simulink subsystem "Plant"  (R2024b)
settings: Solver=VariableStepAuto  StartTime=0.0  StopTime=10.0  RelTol=1e-3
undefined symbols (not defined in the file): fast, GenEff, matches, OutList, rpm2radps, strmatch, TMax
libraries: simulink_extras x1
settings Model: Creator=jhummel  LastModifiedBy=jhummel
settings ModelReferenceCC: EnableRefExpFcnMdlSchedulingChecks=on
settings RTWCC: GPUComputeCapability=3.5

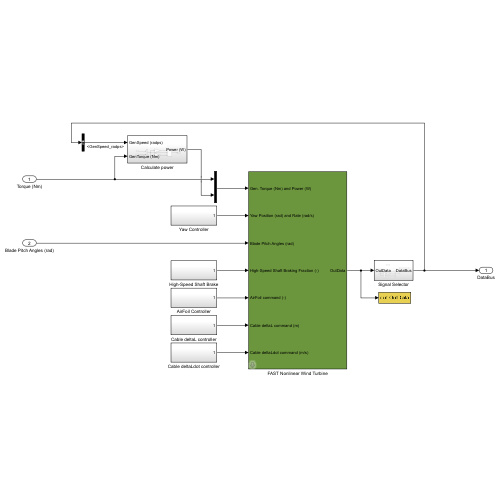
[thumbnail: Simulink's stored preview of the top-level diagram]
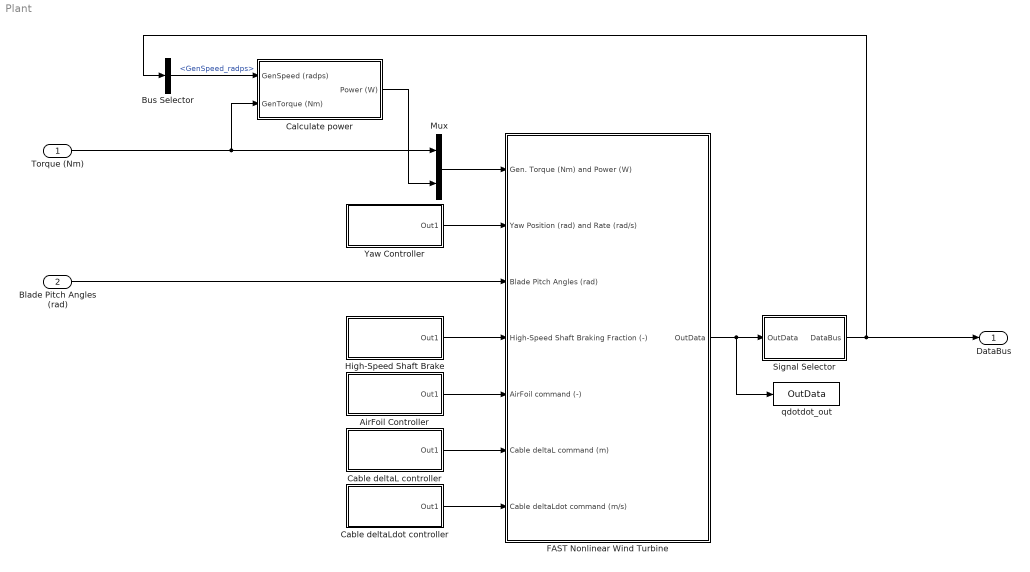
== system Plant ==
  Torque (Nm) : Inport
  Blade Pitch Angles (rad) : Inport  Port=2
  AirFoil Controller : Subsystem
  Bus Selector : BusSelector  OutputSignals=GenSpeed_radps
  Cable deltaL controller : Subsystem
  Cable deltaLdot controller : Subsystem
  Calculate power : Subsystem
  FAST Nonlinear Wind Turbine : Subsystem  mask(FAST Nonlinear Wind Turbine){}
      mask help: This block contains the FAST S-Function.
      mask init:
      | clear FAST_SFunc
  High-Speed Shaft Brake : Subsystem
  Mux : Mux  Inputs=2
  Signal Selector : Subsystem
  Yaw Controller : Subsystem
  qdotdot_out : ToWorkspace  VariableName=OutData  SampleTime=-1
  DataBus : Outport
  wires:
  Yaw Controller/1(Out1) -> FAST Nonlinear Wind Turbine/2(Yaw Position (rad) and Rate (rad/s))
  Mux/1 -> FAST Nonlinear Wind Turbine/1(Gen. Torque (Nm) and Power (W))
  Cable deltaL controller/1(Out1) -> FAST Nonlinear Wind Turbine/6(Cable deltaL command (m))
  High-Speed Shaft Brake/1(Out1) -> FAST Nonlinear Wind Turbine/4(High-Speed Shaft Braking Fraction (-))
  AirFoil Controller/1(Out1) -> FAST Nonlinear Wind Turbine/5(AirFoil command (-))
  Signal Selector/1(DataBus) -> Bus Selector/1, DataBus/1
  Calculate power/1(Power (W)) -> Mux/2
  Torque (Nm)/1 -> Calculate power/2(GenTorque (Nm)), Mux/1
  Cable deltaLdot controller/1(Out1) -> FAST Nonlinear Wind Turbine/7(Cable deltaLdot command (m/s))
  Bus Selector/1 -> Calculate power/1(GenSpeed (radps))  "<GenSpeed_radps>"
  FAST Nonlinear Wind Turbine/1(OutData) -> Signal Selector/1(OutData), qdotdot_out/1
  Blade Pitch Angles (rad)/1 -> FAST Nonlinear Wind Turbine/3(Blade Pitch Angles (rad))

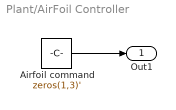
== system Plant/AirFoil Controller ==
  Airfoil command : Constant  Value=zeros(1,3)'
  Out1 : Outport
  wires:
  Airfoil command/1 -> Out1/1

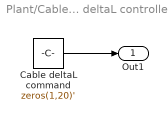
== system Plant/Cable deltaL controller ==
  Cable deltaL command : Constant  Value=zeros(1,20)'
  Out1 : Outport
  wires:
  Cable deltaL command/1 -> Out1/1

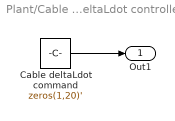
== system Plant/Cable deltaLdot controller ==
  Cable deltaLdot command : Constant  Value=zeros(1,20)'
  Out1 : Outport
  wires:
  Cable deltaLdot command/1 -> Out1/1

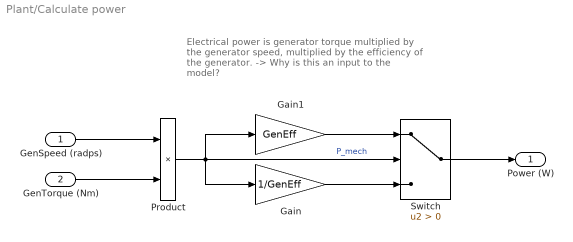
== system Plant/Calculate power ==
  note: Electrical power is generator torque multiplied by the generator speed, multiplied by the efficiency of the generator.
      | -> Why is this an input to the model?
  GenSpeed (radps) : Inport
  GenTorque (Nm) : Inport  Port=2
  Gain : Gain  Gain=1/GenEff
  Gain1 : Gain  Gain=GenEff
  Product : Product
  Switch : Switch  Criteria=u2 > Threshold  SaturateOnIntegerOverflow=off  InputSameDT=off
  Power (W) : Outport
  wires:
  Gain/1 -> Switch/3
  Product/1 -> Switch/2, Gain/1, Gain1/1  "P_mech"
  Gain1/1 -> Switch/1
  GenTorque (Nm)/1 -> Product/2
  GenSpeed (radps)/1 -> Product/1
  Switch/1 -> Power (W)/1

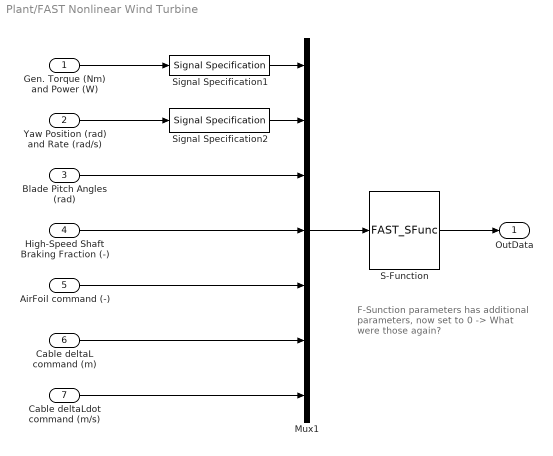
== system Plant/FAST Nonlinear Wind Turbine ==
  note: F-Sunction parameters has additional parameters, now set to 0 -> What were those again?
  Gen. Torque (Nm) and Power (W) : Inport
  Yaw Position (rad) and Rate (rad/s) : Inport  Port=2
  Blade Pitch Angles (rad) : Inport  Port=3
  High-Speed Shaft Braking Fraction (-) : Inport  Port=4
  AirFoil command (-) : Inport  Port=5
  Cable deltaL command (m) : Inport  Port=6
  Cable deltaLdot command (m/s) : Inport  Port=7
  Mux1 : Mux  Inputs=7
  S-Function : S-Function  FunctionName=FAST_SFunc  Parameters=fullfile(fast.FAST_directory, fast.FAST_InputFile), TMax, 0  SFunctionDeploymentMode=off  EnableBusSupport=off
  Signal Specification1 : SignalSpecification  OutDataTypeStr=double  Dimensions=2
  Signal Specification2 : SignalSpecification  OutDataTypeStr=double  Dimensions=2
  OutData : Outport
  wires:
  S-Function/1 -> OutData/1
  Gen. Torque (Nm) and Power (W)/1 -> Signal Specification1/1
  Cable deltaLdot command (m/s)/1 -> Mux1/7
  AirFoil command (-)/1 -> Mux1/5
  Cable deltaL command (m)/1 -> Mux1/6
  Signal Specification2/1 -> Mux1/2
  Mux1/1 -> S-Function/1
  Signal Specification1/1 -> Mux1/1
  Blade Pitch Angles (rad)/1 -> Mux1/3
  High-Speed Shaft Braking Fraction (-)/1 -> Mux1/4
  Yaw Position (rad) and Rate (rad/s)/1 -> Signal Specification2/1

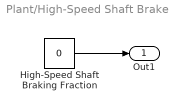
== system Plant/High-Speed Shaft Brake ==
  High-Speed Shaft Braking Fraction : Constant  Value=0
  Out1 : Outport
  wires:
  High-Speed Shaft Braking Fraction/1 -> Out1/1

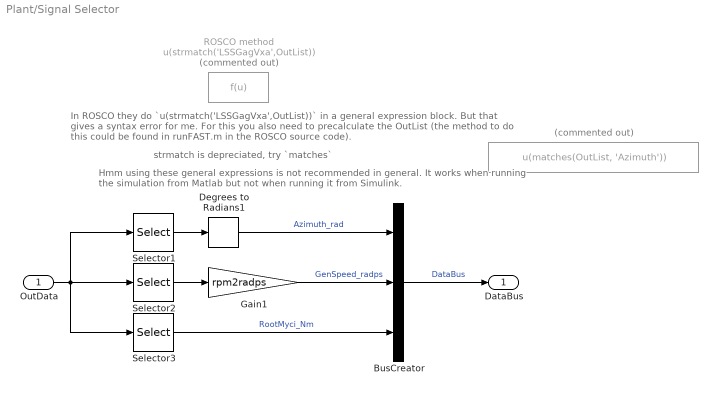
== system Plant/Signal Selector ==
  note: Hmm using these general expressions is not recommended in general. It works when running the simulation from Matlab but not when running it from Simulink.
  note: strmatch is depreciated, try `matches`
  note: In ROSCO they do `u(strmatch('LSSGagVxa',OutList))` in a general expression block. But that gives a syntax error for me. For this you also need to precalculate the OutList (the method to do this could be found in runFAST.m in the ROSCO source code).
  OutData : Inport
  " " : Fcn  Commented=on  Expr=u(matches(OutList, 'Azimuth'))
  BusCreator : BusCreator  Inputs=3
  Degrees to Radians1 : simulink_extras/Transformations/Degrees to Radians
  Gain1 : Gain  Gain=rpm2radps
  ROSCO method : Fcn  Commented=on  Expr=u(strmatch('LSSGagVxa',OutList))
  Selector1 : Selector  InputPortWidth=FAST_indexing.n_vars  IndexOptions=Index vector (dialog)  Indices=FAST_indexing.Azimuth  OutputSizes=1
  Selector2 : Selector  InputPortWidth=FAST_indexing.n_vars  IndexOptions=Index vector (dialog)  Indices=FAST_indexing.GenSpeed  OutputSizes=1
  Selector3 : Selector  InputPortWidth=FAST_indexing.n_vars  IndexOptions=Index vector (dialog)  Indices=FAST_indexing.RootMyci  OutputSizes=1
  DataBus : Outport
  wires:
  Selector2/1 -> Gain1/1
  Degrees to Radians1/1 -> BusCreator/1  "Azimuth_rad"
  Gain1/1 -> BusCreator/2  "GenSpeed_radps"
  Selector3/1 -> BusCreator/3  "RootMyci_Nm"
  BusCreator/1 -> DataBus/1  "DataBus"
  OutData/1 -> Selector3/1, Selector2/1, Selector1/1
  Selector1/1 -> Degrees to Radians1/1

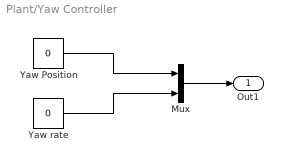
== system Plant/Yaw Controller ==
  Mux : Mux  Inputs=2
  Yaw Position : Constant  Value=0
  Yaw rate : Constant  Value=0
  Out1 : Outport
  wires:
  Mux/1 -> Out1/1
  Yaw Position/1 -> Mux/1
  Yaw rate/1 -> Mux/2
